simulink model "bpsk_rx4_root_raised_cosine_matched_filter"  (R2020b)
settings: Solver=VariableStepAuto  StartTime=0.0  StopTime=1000  RelTol=1e-3
libraries: dsp_blocks x7
settings Model: Creator=hp  LastModifiedBy=hp

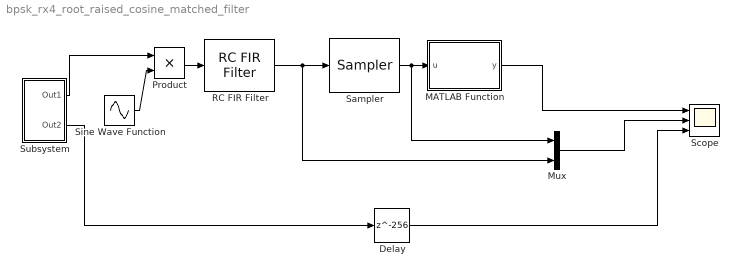
== system bpsk_rx4_root_raised_cosine_matched_filter ==
  Delay : Delay  DelayLength=256
  MATLAB Function : MATLAB Function  TreatAsAtomicUnit=on
  Mux : Mux  Inputs=2
  Product : Product
  RC FIR Filter : dsp_blocks/Filters/RC FIR Filter  period=50  beta=0.5  root=on  filt_len=512  win_type=on
  Sampler : dsp_blocks/Conversions/Sampler  offset=512  samp_period=50
  Scope : Scope  NumInputPorts=3
  Sine Wave Function : Sin  Amplitude=2  Frequency=2*pi*0.1  SampleTime=0
  Subsystem : Subsystem
  wires:
  Subsystem/1(Out1) -> Product/1
  Subsystem/2(Out2) -> Delay/1
  Sine Wave Function/1 -> Product/2
  Product/1 -> RC FIR Filter/1
  RC FIR Filter/1 -> Mux/2, Sampler/1
  Sampler/1 -> MATLAB Function/1(u), Mux/1
  MATLAB Function/1(y) -> Scope/1
  Mux/1 -> Scope/2
  Delay/1 -> Scope/3

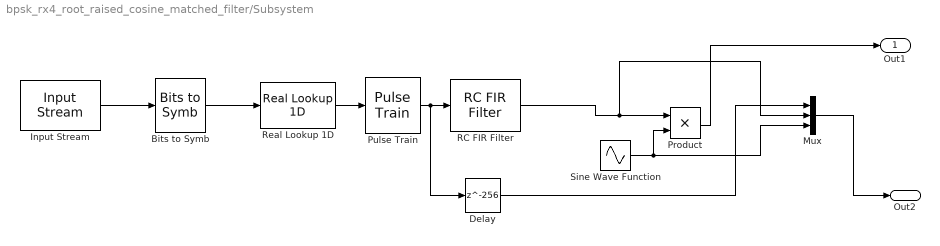
== system bpsk_rx4_root_raised_cosine_matched_filter/Subsystem ==
  Bits to Symb : dsp_blocks/Conversions/Bits to Symb
  Delay : Delay  DelayLength=256
  Input Stream : dsp_blocks/Sources//Sinks/Input Stream  period=50  width=1  fname=rand.mat
  Mux : Mux  Inputs=3
  Product : Product
  Pulse Train : dsp_blocks/Conversions/Pulse Train  period=50
  RC FIR Filter : dsp_blocks/Filters/RC FIR Filter  period=50  beta=0.5  root=on  filt_len=512  win_type=on
  Real Lookup 1D : dsp_blocks/Conversions/Real Lookup 1D  table=[-1 1]
  Sine Wave Function : Sin  Frequency=2*pi*0.1  SampleTime=0
  Out1 : Outport
  Out2 : Outport  Port=2
  wires:
  Real Lookup 1D/1 -> Pulse Train/1
  Pulse Train/1 -> Delay/1, RC FIR Filter/1
  Product/1 -> Out1/1
  RC FIR Filter/1 -> Mux/2, Product/1
  Sine Wave Function/1 -> Mux/3, Product/2
  Bits to Symb/1 -> Real Lookup 1D/1
  Input Stream/1 -> Bits to Symb/1
  Delay/1 -> Mux/1
  Mux/1 -> Out2/1

== matlab function bpsk_rx4_root_raised_cosine_matched_filter/MATLAB Function ==
  data: u input; y output
function y = fcn(u)
if (u > 0)
    y = 1;
else
    y = 0;
end
